simulink model "startingsequencee"  (R2025a)
settings: Solver=VariableStepAuto  StartTime=0.0  StopTime=10.0  RelTol=1e-3
libraries: simulink x1
settings Model: Creator=HP  LastModifiedBy=HP

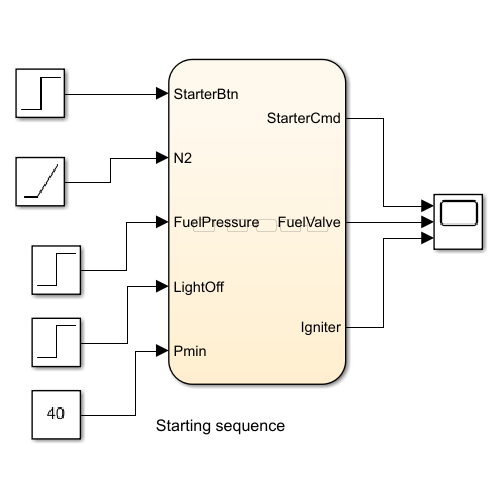
[thumbnail: Simulink's stored preview of the top-level diagram]
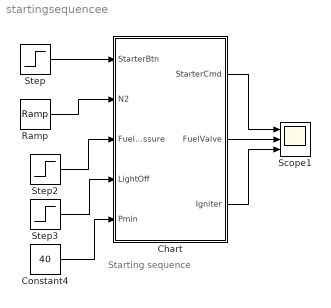
== system startingsequencee ==
  note: Starting sequence
  Chart : Stateflow chart  TreatAsAtomicUnit=on
  Constant4 : Constant  Value=40
  Ramp : simulink/Sources/Ramp  slope=20  start=0  InitialOutput=0
  Scope1 : Scope  NumInputPorts=3
      settings: ActiveDisplayYMinimum=-143.1192654934672  ActiveDisplayYMaximum=252.10003371530803
  Step : Step  SampleTime=0
  Step2 : Step  Time=2  After=30  SampleTime=0
  Step3 : Step  Time=3  SampleTime=0
  wires:
  Chart/2(FuelValve) -> Scope1/2
  Step/1 -> Chart/1(StarterBtn)
  Step3/1 -> Chart/4(LightOff)
  Chart/1(StarterCmd) -> Scope1/1
  Chart/3(Igniter) -> Scope1/3
  Constant4/1 -> Chart/5(Pmin)
  Step2/1 -> Chart/3(FuelPressure)
  Ramp/1 -> Chart/2(N2)

== stateflow chart startingsequencee/Chart ==
  state during_1
    StarterCmd = 0;
    FuelValve = 0;
    Igniter = 0;
  state during_2
    StarterCmd = 1;
    FuelValve = 0;
    Igniter = 0;
  state during_3
    StarterCmd = 1;
    FuelValve = 1;
    Igniter = 1;
  state during_4
    StarterCmd = 1;
    FuelValve = 1;
    Igniter = 0;
  state during_5
    StarterCmd = 0;
    FuelValve = 1;
    Igniter = 0;
  (default) -> during_1
  during_1 -> during_2 : [StarterBtn == 1]
  during_2 -> during_3 : [N2 >= 40 && FuelPressure > Pmin]
  during_3 -> during_4 : [LightOff == 1]
  during_4 -> during_5 : [N2 >= 60]
  data: StarterCmd output; StarterBtn input; N2 input; FuelPressure input; LightOff input; FuelValve output; Igniter output; Pmin input
